simulink model "hades_sim"  (R2018b)
settings: Solver=VariableStepDiscrete  StartTime=0.0  StopTime=10  RelTol=1e-3
settings Model: Creator=vivek  LastModifiedBy=vivek

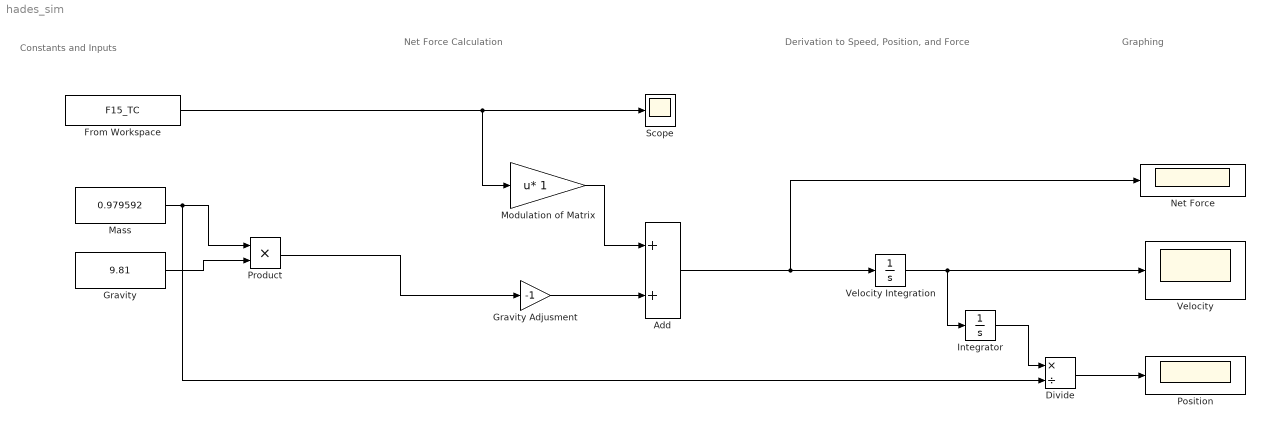
== system hades_sim ==
  note: Graphing
  note: Derivation to Speed, Position, and Force
  note: Net Force Calculation
  note: Constants and Inputs
  Add : Sum
  Divide : Product  Inputs=*/
  From Workspace : FromWorkspace  VariableName=F15_TC  OutDataTypeStr=double  SampleTime=0  OutputAfterFinalValue=Setting to zero
  "Gravity " : Constant  Value=9.81
  "Gravity Adjusment " : Gain  Gain=-1
  Integrator : Integrator  LimitOutput=on  LowerSaturationLimit=0
  "Mass " : Constant  Value=0.979592
  "Modulation of Matrix " : Gain  Multiplication=Matrix(u*K)
  "Net Force " : Scope
  "Position " : Scope
  Product : Product
  Scope : Scope
  "Velocity " : Scope
  "Velocity Integration " : Integrator  LowerSaturationLimit=0
  wires:
  "Mass "/1 -> Divide/2, Product/1
  "Gravity "/1 -> Product/2
  From Workspace/1 -> "Modulation of Matrix "/1, Scope/1
  Product/1 -> "Gravity Adjusment "/1
  "Gravity Adjusment "/1 -> Add/2
  "Modulation of Matrix "/1 -> Add/1
  Add/1 -> "Net Force "/1, "Velocity Integration "/1
  "Velocity Integration "/1 -> Integrator/1, "Velocity "/1
  Integrator/1 -> Divide/1
  Divide/1 -> "Position "/1
